simulink model "sampleModel2049_2"  (R2023a)
settings: Solver=VariableStepAuto  StartTime=0.0  StopTime=10.0  RelTol=1e-3
libraries: hdlsllib x3, simulink x2
settings Model: Creator=user1  LastModifiedBy=user1

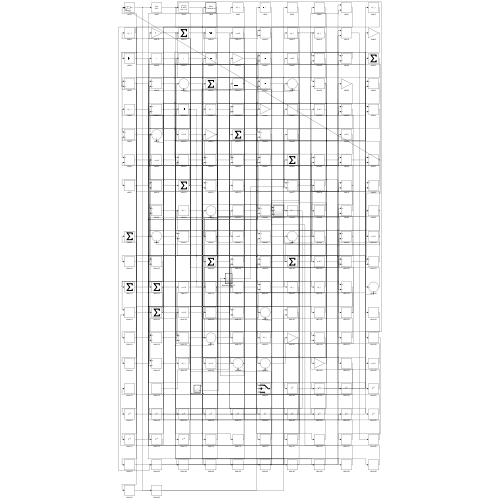
[thumbnail: Simulink's stored preview of the top-level diagram]
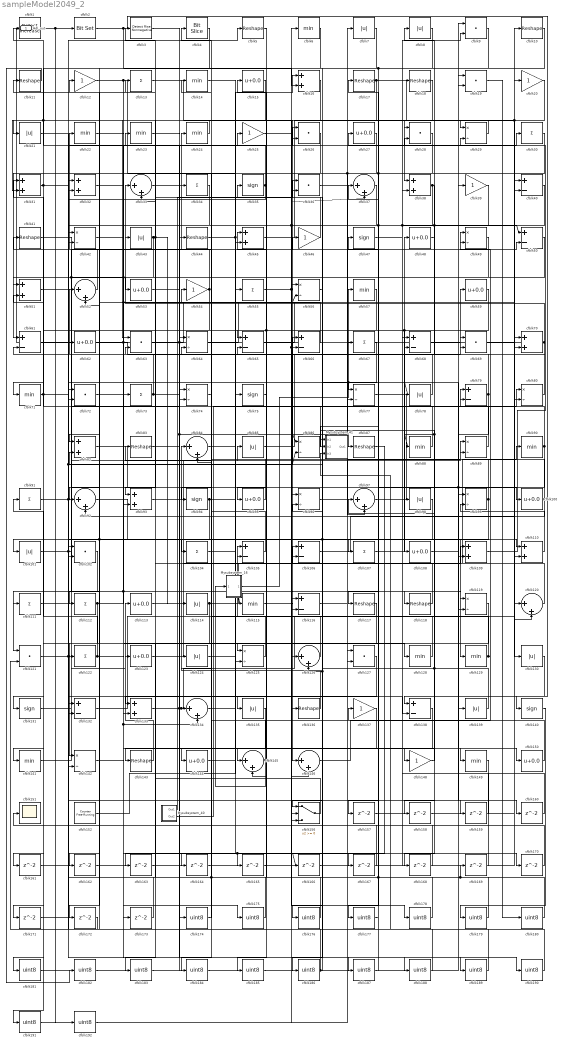
== system sampleModel2049_2 ==
  Mysubsystem_16 : Subsystem  TreatAsAtomicUnit=on  RTWFcnName=Mysubsystem_16
      settings: RTWFcnNameOpts=User specified  RTWFileNameOpts=Use function name
  Mysubsystem_40 : Subsystem  TreatAsAtomicUnit=on  RTWFcnName=Mysubsystem_40
      settings: RTWFcnNameOpts=User specified  RTWFileNameOpts=Use function name
  Mysubsystem_41 : Subsystem  TreatAsAtomicUnit=on  RTWFcnName=Mysubsystem_41
      settings: RTWFcnNameOpts=User specified  RTWFileNameOpts=Use function name
  cfblk1 : simulink/Logic and Bit Operations/Detect Increase  vinit=0.0  OutDataTypeStr=uint8
      settings: LibrarySourceBlock=|
      | hdlsllib/Logic and Bit
      | Operations/Detect
      | Increase
  cfblk{5,10..11,17..18,41,44,83,87,117..118,136,143} (13 alike) : Reshape
  cfblk{15,27,48,53,59,62,95,100,108,113,123,144,150} (13 alike) : Bias  Bias=0.0  SaturateOnIntegerOverflow=off
  cfblk{7..8,21,43,78,85,98,101,114,124,130,135,139} (13 alike) : Abs  OutDataTypeStr=uint8  SaturateOnIntegerOverflow=off
  cfblk{9,19,26,28,36,63,69,72,102,121,127} (11 alike) : DotProduct  OutDataTypeStr=uint8
  cfblk{13,30,34,55,67,73,91,104,107,111..112,122} (12 alike) : Sum  Inputs=+  OutDataTypeStr=uint8
  cfblk{40,50,61,65..66,68,79,105..106,116,132,138} (12 alike) : Sum  Inputs=+-  OutDataTypeStr=uint8
  cfblk{16,31..32,38,45,51,70,82,93,109..110,133} (12 alike) : Sum  OutDataTypeStr=uint8
  cfblk{6,14,22..24,57,71,88,90,115,128..129,141,149} (14 alike) : MinMax  OutDataTypeStr=uint8
  cfblk{29,42,49,56,64,74,77,80,86,89,96,99,119,125,142} (15 alike) : Product  Inputs=*/  OutDataTypeStr=uint8  RndMeth=Zero  SaturateOnIntegerOverflow=on
  cfblk{12,20,25,39,46,54,137,148} (8 alike) : Gain  OutDataTypeStr=uint8
  cfblk{33,37,52,84,92,97,120,126,134,145..146} (11 alike) : Sum  Inputs=|++  OutDataTypeStr=uint8
  cfblk{35,47,75,94,131,140} (6 alike) : Signum
  cfblk151 : Scope
  cfblk152 : hdlsllib/Sources/Counter Free-Running  NumBits=16  tsamp=-1
  cfblk156 : Switch  OutDataTypeStr=uint8  SaturateOnIntegerOverflow=off  InputSameDT=off
  cfblk{157..173} (17 alike) : Delay  SampleTime=1
  cfblk{174..192} (19 alike) : DataTypeConversion  OutDataTypeStr=uint8  SaturateOnIntegerOverflow=off  RndMeth=Floor
  cfblk2 : simulink/Logic and Bit Operations/Bit Set  iBit=0
      settings: LibrarySourceBlock=|
      | hdlsllib/Logic and Bit
      | Operations/Bit Set
  cfblk3 : hdlsllib/Logic and Bit Operations/Detect Rise Nonnegative  vinit=0  OutDataTypeStr=uint8
  cfblk4 : hdlsllib/Logic and Bit Operations/Bit Slice  lidx=7  ridx=0
  Hdl_out : Outport  OutDataTypeStr=uint8
  wires:
  cfblk54/1 -> cfblk24/1, cfblk93/2
  cfblk70/1 -> cfblk33/1, cfblk65/2, Hdl_out/1
  cfblk23/1 -> cfblk128/1
  cfblk109/1 -> cfblk27/1
  cfblk139/1 -> cfblk97/1, cfblk82/2
  cfblk146/1 -> cfblk90/1
  cfblk24/1 -> cfblk63/1
  cfblk74/1 -> cfblk4/1
  cfblk107/1 -> cfblk48/1
  cfblk15/1 -> cfblk31/2, cfblk181/1
  cfblk45/1 -> cfblk29/1
  cfblk149/1 -> cfblk151/1
  cfblk97/1 -> cfblk79/1
  cfblk26/1 -> cfblk61/1
  cfblk13/1 -> cfblk146/1
  cfblk101/1 -> cfblk46/1, cfblk190/1
  cfblk143/1 -> cfblk113/1
  cfblk125/1 -> cfblk105/1
  cfblk2/1 -> cfblk140/1, cfblk16/2
  cfblk51/1 -> cfblk100/1
  cfblk61/1 -> cfblk116/1
  cfblk141/1 -> cfblk85/1
  cfblk41/1 -> cfblk139/1, cfblk73/1
  cfblk33/1 -> cfblk74/2
  cfblk39/1 -> cfblk117/1, cfblk104/1
  cfblk114/1 -> cfblk39/1, cfblk133/1
  cfblk52/1 -> cfblk22/1
  cfblk66/1 -> cfblk11/1
  cfblk136/1 -> cfblk84/1
  cfblk128/1 -> cfblk45/1
  cfblk137/1 -> cfblk186/1
  cfblk59/1 -> cfblk135/1, cfblk94/1, cfblk108/1
  cfblk96/1 -> cfblk98/1
  cfblk40/1 -> cfblk88/1, cfblk148/1, cfblk144/1, cfblk156/3
  cfblk82/1 -> cfblk96/1
  cfblk18/1 -> cfblk38/1
  cfblk38/1 -> cfblk102/2, cfblk158/1
  cfblk123/1 -> cfblk89/1
  cfblk71/1 -> cfblk5/1, cfblk141/1
  cfblk8/1 -> cfblk56/1
  cfblk100/1 -> cfblk14/1, cfblk92/2
  cfblk150/1 -> cfblk83/1
  cfblk92/1 -> cfblk129/1
  cfblk135/1 -> cfblk145/1
  cfblk99/1 -> cfblk136/1, cfblk132/2, cfblk62/1
  cfblk84/1 -> cfblk87/1
  cfblk47/1 -> cfblk50/1, cfblk9/2
  cfblk28/1 -> cfblk77/2, cfblk164/1
  cfblk145/1 -> Mysubsystem_16/1(In1), cfblk61/2
  cfblk152/1 -> cfblk49/1
  cfblk35/1 -> cfblk32/2, cfblk1/1
  cfblk133/1 -> cfblk80/2, cfblk134/1, cfblk30/1
  cfblk102/1 -> cfblk121/1
  cfblk86/1 -> cfblk15/1
  cfblk91/1 -> cfblk34/1, cfblk138/2
  cfblk46/1 -> cfblk12/1
  cfblk25/1 -> cfblk178/1
  cfblk30/1 -> Mysubsystem_41/1(In1), cfblk92/1
  cfblk89/1 -> cfblk47/1
  cfblk78/1 -> cfblk52/1
  cfblk126/1 -> cfblk84/2
  cfblk29/1 -> cfblk28/1
  cfblk121/1 -> cfblk86/2, cfblk26/2, cfblk159/1
  cfblk27/1 -> cfblk71/1
  cfblk124/1 -> cfblk45/2
  cfblk43/1 -> cfblk72/2, cfblk133/2, cfblk114/1, cfblk93/1
  cfblk50/1 -> cfblk101/1
  cfblk17/1 -> cfblk120/1, cfblk53/1
  cfblk7/1 -> cfblk112/1
  cfblk138/1 -> cfblk143/1
  cfblk75/1 -> cfblk95/1
  cfblk111/1 -> cfblk119/1
  cfblk21/1 -> cfblk110/1
  cfblk53/1 -> cfblk150/1
  cfblk32/1 -> cfblk125/1
  cfblk1/1 -> cfblk2/1, cfblk192/1
  cfblk115/1 -> cfblk116/2
  cfblk95/1 -> cfblk41/1
  cfblk117/1 -> cfblk131/1
  cfblk36/1 -> cfblk97/2
  cfblk79/1 -> cfblk8/1, cfblk119/2
  cfblk20/1 -> cfblk70/2, cfblk65/1
  cfblk44/1 -> cfblk36/1, cfblk167/1
  cfblk90/1 -> cfblk107/1, cfblk109/2, cfblk68/2
  cfblk110/1 -> cfblk99/2
  cfblk31/1 -> cfblk77/1, cfblk78/1, cfblk51/1
  cfblk116/1 -> cfblk89/2
  cfblk132/1 -> cfblk18/1
  cfblk48/1 -> cfblk138/1
  cfblk118/1 -> cfblk37/1
  cfblk62/1 -> cfblk56/2, cfblk26/1, cfblk69/2
  cfblk129/1 -> cfblk96/2, cfblk49/2
  cfblk88/1 -> cfblk51/2
  cfblk119/1 -> cfblk142/1
  cfblk63/1 -> cfblk10/1, cfblk110/2
  cfblk134/1 -> cfblk75/1
  cfblk112/1 -> cfblk29/2, cfblk115/1, cfblk142/2
  cfblk19/1 -> cfblk180/1
  cfblk113/1 -> cfblk109/1
  cfblk68/1 -> cfblk59/1
  cfblk144/1 -> cfblk106/1
  cfblk131/1 -> cfblk123/1
  cfblk85/1 -> cfblk69/1
  cfblk55/1 -> cfblk118/1, cfblk37/2
  cfblk72/1 -> cfblk134/2, cfblk187/1
  cfblk65/1 -> cfblk9/1
  cfblk80/1 -> cfblk28/2
  cfblk69/1 -> cfblk130/1
  cfblk93/1 -> cfblk66/1
  cfblk73/1 -> cfblk86/1, cfblk125/2, cfblk31/1
  cfblk12/1 -> cfblk55/1, cfblk149/1
  cfblk106/1 -> cfblk20/1
  cfblk105/1 -> cfblk64/2
  cfblk142/1 -> cfblk165/1, cfblk166/1
  cfblk10/1 -> cfblk82/1, cfblk177/1
  cfblk94/1 -> cfblk50/2, cfblk111/1
  cfblk156/1 -> cfblk23/1
  cfblk122/1 -> cfblk91/1, cfblk175/1
  cfblk56/1 -> cfblk126/1
  cfblk9/1 -> cfblk156/1
  cfblk77/1 -> cfblk79/2
  cfblk98/1 -> cfblk122/1, cfblk171/1
  cfblk120/1 -> cfblk13/1
  cfblk16/1 -> cfblk156/2, cfblk66/2
  cfblk4/1 -> cfblk21/1
  cfblk64/1 -> cfblk40/2
  cfblk104/1 -> cfblk16/1
  cfblk87/1 -> cfblk157/1
  cfblk157/1 -> cfblk40/1
  cfblk158/1 -> cfblk70/1
  cfblk159/1 -> cfblk99/1
  cfblk108/1 -> cfblk160/1
  cfblk160/1 -> cfblk68/1
  cfblk57/1 -> cfblk161/1
  cfblk161/1 -> cfblk74/1
  cfblk37/1 -> cfblk162/1
  cfblk162/1 -> cfblk38/2
  cfblk163/1 -> cfblk64/1
  cfblk164/1 -> cfblk146/2
  cfblk165/1 -> cfblk106/2
  cfblk166/1 -> cfblk120/2
  cfblk167/1 -> cfblk105/2
  cfblk130/1 -> cfblk168/1
  cfblk168/1 -> cfblk102/1
  cfblk169/1 -> cfblk63/2
  cfblk14/1 -> cfblk170/1
  cfblk170/1 -> cfblk33/2
  cfblk171/1 -> cfblk132/1
  cfblk34/1 -> cfblk172/1
  cfblk172/1 -> cfblk121/2
  cfblk22/1 -> cfblk173/1
  cfblk173/1 -> cfblk52/2
  cfblk3/1 -> cfblk174/1
  cfblk174/1 -> cfblk124/1
  cfblk175/1 -> cfblk3/1
  cfblk67/1 -> cfblk176/1
  cfblk176/1 -> cfblk72/1
  cfblk177/1 -> cfblk67/1
  cfblk178/1 -> cfblk43/1, cfblk54/1
  cfblk140/1 -> cfblk179/1
  cfblk179/1 -> cfblk25/1
  cfblk180/1 -> cfblk145/2, cfblk17/1, cfblk169/1
  cfblk181/1 -> cfblk19/1
  cfblk11/1 -> cfblk182/1
  cfblk182/1 -> cfblk19/2
  cfblk127/1 -> cfblk183/1
  cfblk183/1 -> cfblk44/1
  cfblk49/1 -> cfblk184/1
  cfblk184/1 -> cfblk127/1
  cfblk5/1 -> cfblk185/1
  cfblk185/1 -> cfblk127/2
  cfblk186/1 -> cfblk126/2, cfblk36/2, cfblk32/1
  cfblk187/1 -> cfblk137/1
  cfblk42/1 -> cfblk188/1
  cfblk83/1 -> cfblk189/1
  cfblk189/1 -> cfblk42/1
  cfblk190/1 -> cfblk42/2
  cfblk6/1 -> cfblk191/1
  cfblk191/1 -> cfblk7/1
  cfblk192/1 -> cfblk6/1
  Mysubsystem_16/1(Out1) -> cfblk57/1
  Mysubsystem_40/1(Out1) -> cfblk35/1
  Mysubsystem_40/2(Out2) -> cfblk80/1
  cfblk148/1 -> Mysubsystem_41/2(In2)
  cfblk188/1 -> Mysubsystem_41/3(In3)
  Mysubsystem_41/1(Out1) -> cfblk163/1

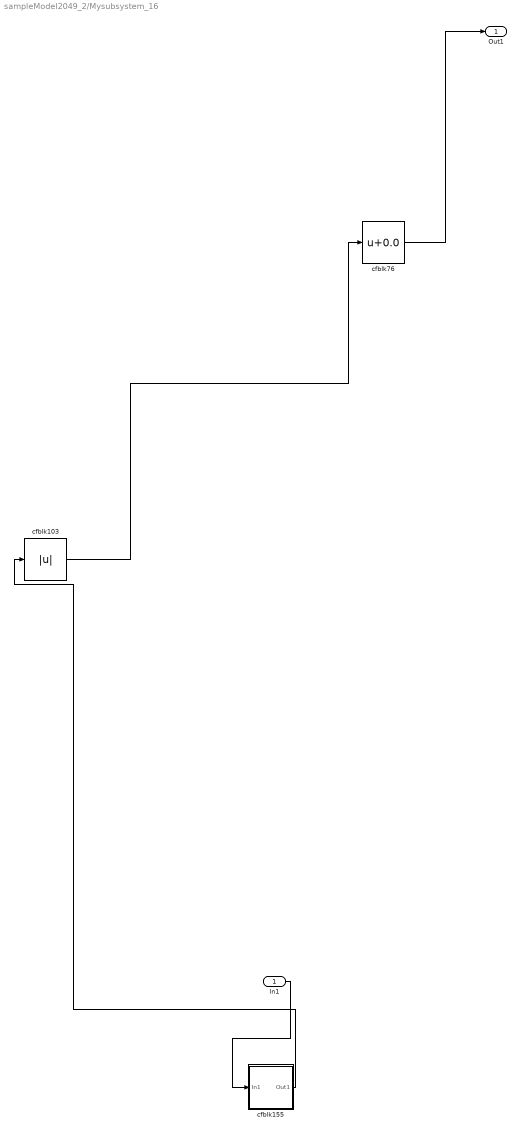
== system sampleModel2049_2/Mysubsystem_16 ==
  In1 : Inport
  cfblk103 : Abs  SaturateOnIntegerOverflow=off
  cfblk155 : Subsystem
      settings: LibrarySourceBlock=|
      | hdlsllib/Ports &
      | Subsystems/Subsystem
  cfblk76 : Bias  Bias=0.0  SaturateOnIntegerOverflow=off
  Out1 : Outport
  wires:
  In1/1 -> cfblk155/1(In1)
  cfblk76/1 -> Out1/1
  cfblk103/1 -> cfblk76/1
  cfblk155/1(Out1) -> cfblk103/1

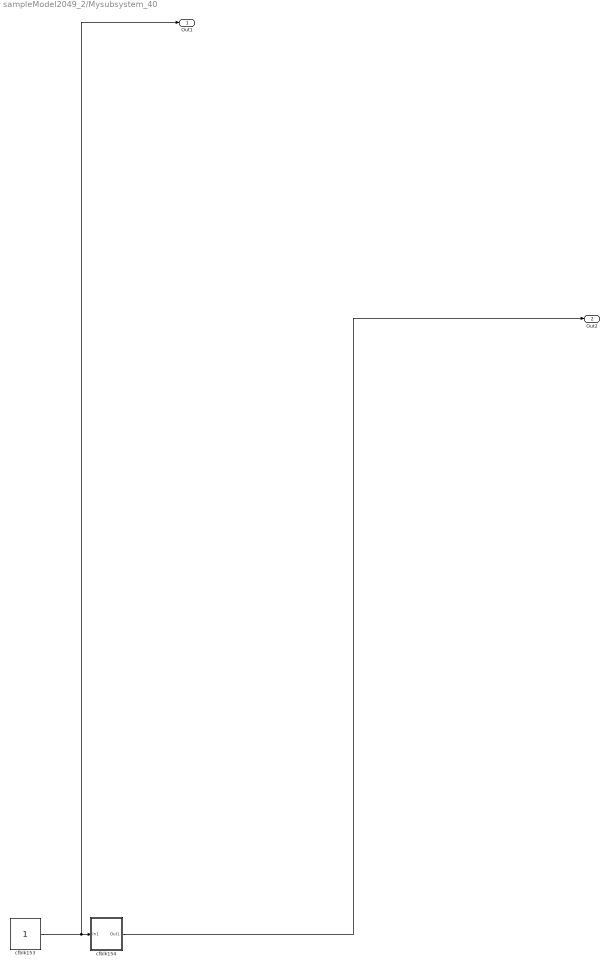
== system sampleModel2049_2/Mysubsystem_40 ==
  cfblk153 : Constant  SampleTime=-1
  cfblk154 : Subsystem
      settings: LibrarySourceBlock=|
      | hdlsllib/Ports &
      | Subsystems/Subsystem
  Out1 : Outport
  Out2 : Outport  Port=2
  wires:
  cfblk153/1 -> Out1/1, cfblk154/1(In1)
  cfblk154/1(Out1) -> Out2/1

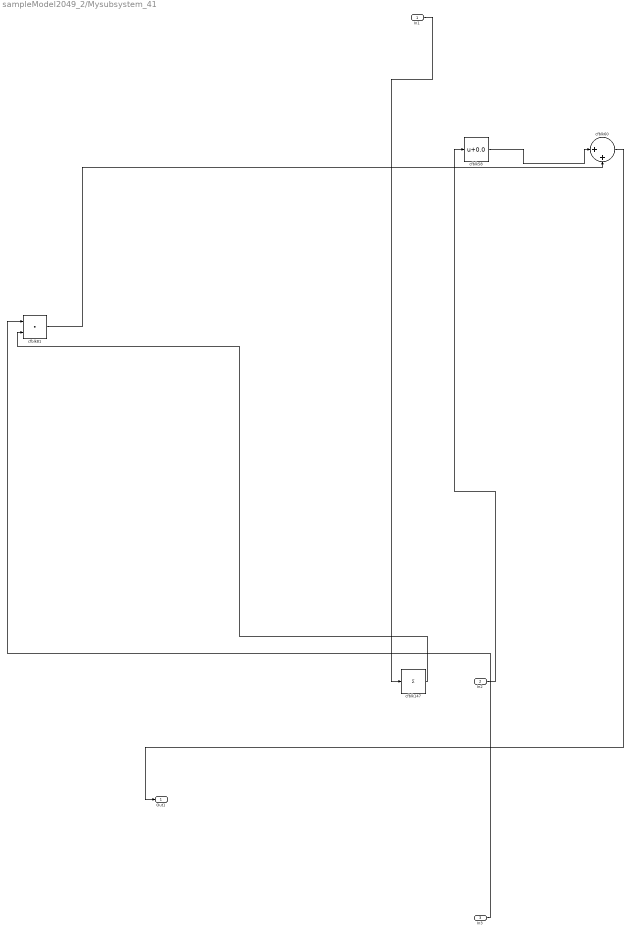
== system sampleModel2049_2/Mysubsystem_41 ==
  In1 : Inport
  In2 : Inport  Port=2
  In3 : Inport  Port=3
  cfblk147 : Sum  Inputs=+
  cfblk58 : Bias  Bias=0.0  SaturateOnIntegerOverflow=off
  cfblk60 : Sum  Inputs=|++
  cfblk81 : DotProduct  OutDataTypeStr=Inherit: Inherit via internal rule
  Out1 : Outport
  wires:
  cfblk58/1 -> cfblk60/1
  cfblk81/1 -> cfblk60/2
  cfblk147/1 -> cfblk81/2
  In3/1 -> cfblk81/1
  cfblk60/1 -> Out1/1
  In2/1 -> cfblk58/1
  In1/1 -> cfblk147/1

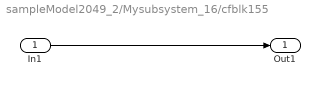
== system sampleModel2049_2/Mysubsystem_16/cfblk155 ==
  In1 : Inport
  Out1 : Outport
  wires:
  In1/1 -> Out1/1

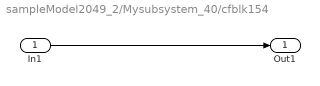
== system sampleModel2049_2/Mysubsystem_40/cfblk154 ==
  In1 : Inport
  Out1 : Outport
  wires:
  In1/1 -> Out1/1
